simulink model "model_free"  (R2024a)
settings: Solver=FixedStepAuto  StartTime=0.0  StopTime=10.0  RelTol=1e-3
model workspace (MAT data in the model file):
  D = 0.006
  I = 0.04472
  Kp = 150
  Kpc = 250
  Kpp = 1600
  N = 17
  Nd = 10
  P = 5000
  Td = 0.005075
  Ti = 1000000
  Ts = 0.005
  alpha = 0.9
undefined symbols (not defined in the file or in its folder): GS, PID
libraries: slpidlib x3, simulink x2
settings Model: Creator=Henrique Mesquita  LastModifiedBy=Henrique Mesquita
settings SolverCC: ConcurrentTasks=on  PositivePriorityOrder=on
settings OptimizationCC: BlockReduction=off  OptimizeBlockIOStorage=off  ReuseModelBlockBuffer=off
settings DebuggingCC: TasksWithSamePriorityMsg=none  UnconnectedInputMsg=warning  UnconnectedOutputMsg=warning  UnconnectedLineMsg=warning
settings HardwareCC: ProdBitPerLong=64  ProdLongLongMode=on  ProdHWDeviceType=Intel->x86-64 (Linux 64)
settings ModelReferenceCC: EnableRefExpFcnMdlSchedulingChecks=on
settings RTWCC: Description=Speedgoat Real-Time Target Machine  SystemTargetFile=speedgoat.tlc  TemplateMakefile=slrealtime_default_tmf  Toolchain=Simulink Real-Time Toolchain  BuildConfiguration=Faster Runs  CodeExecutionProfiling=on  TargetLang=C++  GPUComputeCapability=3.5  DLArmComputeVersion=19.05
settings SimulinkRealTimeTargetCC: InstructionSetFMA=off  LogToMDFFile=off

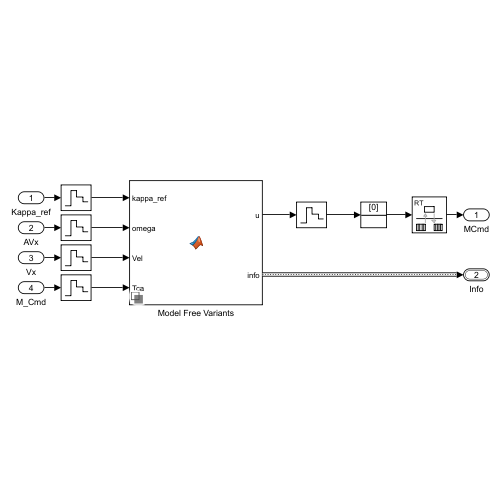
[thumbnail: Simulink's stored preview of the top-level diagram]
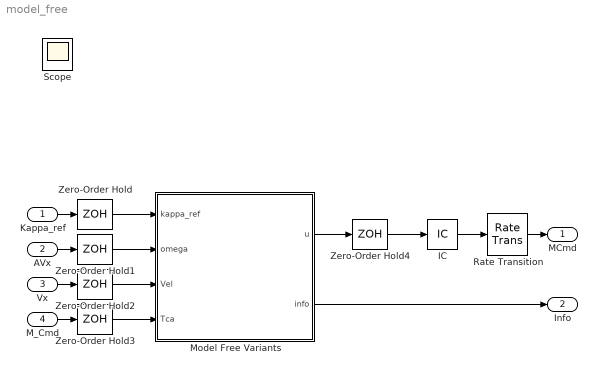
== system model_free ==
  Kappa_ref : Inport
  AVx : Inport  Port=2
  Vx : Inport  Port=3
  M_Cmd : Inport  Port=4
  IC : InitialCondition  Value=0
  Model Free Variants : Subsystem  Variant=on  VariantControlMode=label  VariantControl=Choice  LabelModeActiveChoice=MFC sliding window
  Rate Transition : RateTransition
  Zero-Order Hold{,1..4} (5 alike) : ZeroOrderHold  SampleTime=Ts
  MCmd : Outport
  Info : Outport  Port=2  OutDataTypeStr=Bus: control_info_bus
  Scope : Scope
  wires:
  AVx/1 -> Zero-Order Hold1/1
  IC/1 -> Rate Transition/1
  Vx/1 -> Zero-Order Hold2/1
  M_Cmd/1 -> Zero-Order Hold3/1
  Rate Transition/1 -> MCmd/1
  Kappa_ref/1 -> Zero-Order Hold/1
  Zero-Order Hold4/1 -> IC/1
  Zero-Order Hold/1 -> Model Free Variants/1(kappa_ref)
  Zero-Order Hold1/1 -> Model Free Variants/2(omega)
  Zero-Order Hold2/1 -> Model Free Variants/3(Vel)
  Zero-Order Hold3/1 -> Model Free Variants/4(Tca)
  Model Free Variants/1(u) -> Zero-Order Hold4/1
  Model Free Variants/2(info) -> Info/1

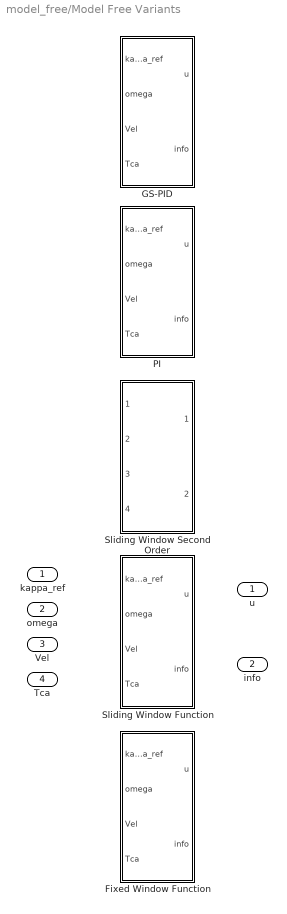
== system model_free/Model Free Variants ==
  kappa_ref : Inport
  omega : Inport  Port=2
  Vel : Inport  Port=3
  Tca : Inport  Port=4
  Fixed Window Function : MATLAB Function  TreatAsAtomicUnit=on  VariantControl=Choice_2
  GS-PID : Subsystem  VariantControl=GS-PID
  PI : Subsystem  VariantControl=PID
  Sliding Window Function : MATLAB Function  TreatAsAtomicUnit=on  VariantControl=MFC sliding window
  Sliding Window Second Order : ModelReference  ModelNameDialog=Sliding_Window_Second_Order  SimulationMode=Normal  VariantControl=Choice  ModelReferenceVersion=1.164
  u : Outport
  info : Outport  Port=2

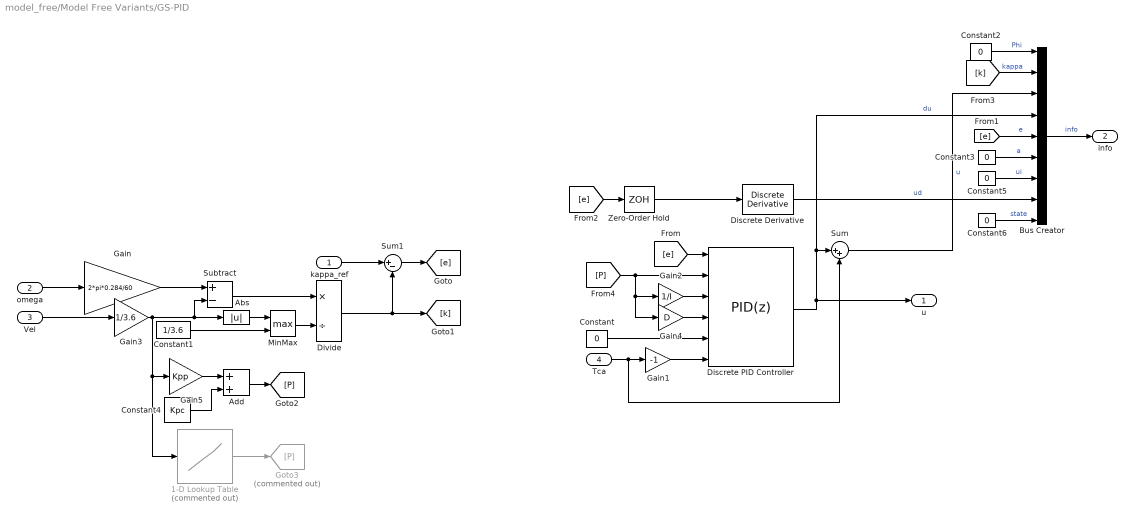
== system model_free/Model Free Variants/GS-PID ==
  kappa_ref : Inport
  omega : Inport  Port=2
  Vel : Inport  Port=3
  Tca : Inport  Port=4
  1-D Lookup Table : Lookup_n-D  Commented=on  NumberOfTableDimensions=1  BreakpointsForDimension1=[0:2]  Table=[Kpc,Kpc,Kpc+Kpp]  InternalRulePriority=Speed  RndMeth=Simplest
  Abs : Abs  SaturateOnIntegerOverflow=off
  Add : Sum
  Bus Creator : BusCreator  Inputs=9  OutDataTypeStr=Bus: control_info_bus
      settings: InheritFromInputs=off
  Constant{,2..3,5..6} (5 alike) : Constant  Value=0  SampleTime=Ts
  Constant1 : Constant  Value=1/3.6
  Constant4 : Constant  Value=Kpc
  Discrete Derivative : simulink/Discrete/Discrete Derivative  gainval=P*D  ICPrevScaledInput=0.0  OutMin=[]  OutMax=[]  OutDataType=fixdt(1, 16)  OutScaling=2^-10  DoSatur=off
  Discrete PID Controller : slpidlib/PID Controller  Controller=PID  Form=Parallel  TimeDomain=Discrete-time  UseExternalTs=off  SampleTime=Ts  IntegratorMethod=Trapezoidal  FilterMethod=Forward Euler  ControllerParametersSource=external  P=P  I=P/I  UseKiTs=off  D=P*D  UseExternalDerivativeSource=off  N=100  UseFilter=off  TunerSelectOption=Transfer Function Based (PID Tuner App)  InitialConditionSource=internal  InitialConditionForIntegrator=0  InitialConditionForFilter=0  DifferentiatorICPrevScaledInput=0  ExternalReset=none  TrackingMode=off  Kt=1  LimitOutput=on  SatLimitsSource=external  UpperSaturationLimit=inf  LowerSaturationLimit=-inf  LinearizeAsGain=off  AntiWindupMode=clamping  Kb=1  LimitIntegrator=off  UpperIntegratorSaturationLimit=inf  LowerIntegratorSaturationLimit=-inf  POutMin=[]  POutMax=[]  IOutMin=[]  IOutMax=[]  DOutMin=[]  DOutMax=[]  NOutMin=[]  NOutMax=[]  SumOutMin=[]  SumOutMax=[]  SaturationOutMin=[]  SaturationOutMax=[]  PParamMin=[]  PParamMax=[]  IParamMin=[]  IParamMax=[]  DParamMin=[]  DParamMax=[]  NParamMin=[]  NParamMax=[]  KbParamMin=[]  KbParamMax=[]  KtParamMin=[]  KtParamMax=[]  KbOutMin=[]  KbOutMax=[]  KtOutMin=[]  KtOutMax=[]  IntegratorOutMin=[]  IntegratorOutMax=[]  FilterOutMin=[]  FilterOutMax=[]  SumI1OutMin=[]  SumI1OutMax=[]  SumI2OutMin=[]  SumI2OutMax=[]  SumI3OutMin=[]  SumI3OutMax=[]  SumI4OutMin=[]  SumI4OutMax=[]  SumDOutMin=[]  SumDOutMax=[]  DifferentiatorOutMin=[]  DifferentiatorOutMax=[]  FilterDiffOutCoefMin=[]  FilterDiffOutCoefMax=[]  ReciprocalOutMin=[]  ReciprocalOutMax=[]  SumDenOutMin=[]  SumDenOutMax=[]  SumNumOutMin=[]  SumNumOutMax=[]  DivideOutMin=[]  DivideOutMax=[]  UdiffTsProdOutMin=[]  UdiffTsProdOutMax=[]  NTsProdOutMin=[]  NTsProdOutMax=[]  UintegralTsProdOutMin=[]  UintegralTsProdOutMax=[]  UngainTsProdOutMin=[]  UngainTsProdOutMax=[]  ClampingZeroOutDataTypeStr=Inherit: Inherit via back propagation  ClampingZeroOutMin=[]  ClampingZeroOutMax=[]  FilterDenConstantOutDataTypeStr=Inherit: Inherit via back propagation  FilterDenConstantOutMin=[]  FilterDenConstantOutMax=[]  PCopyOutDataTypeStr=Inherit: Inherit via back propagation  PCopyOutMin=[]  PCopyOutMax=[]  NCopyOutDataTypeStr=Inherit: Inherit via back propagation  NCopyOutMin=[]  NCopyOutMax=[]  IntegratorContinuousStateAttributes=''  IntegratorStateMustResolveToSignalObject=off  IntegratorRTWStateStorageClass=Auto  FilterContinuousStateAttributes=''  FilterStateMustResolveToSignalObject=off  FilterRTWStateStorageClass=Auto  ParallelPVariant=ExternalParameters  IdealPVariant=Disabled  IVariant=ExternalParameters  DVariant=ExternalParameters  IntegratorVariant=Discrete  SatVariant=External  AWVariant=DiscClampingParallel  PCopyVariant=Disabled  TRVariant=Disabled  FdbkBlocksVariant=Feedback  IdealPFdbkVariant=Passthrough  SatFdbkVariant=Passthrough  DerivativeFilterVariant=Differentiator  NVariant=Passthrough  NCopyVariant=Disabled_SignalSpec  FilterICVariant=InternalICsDifferentiator  IntegratorICVariant=InternalICs  ExternalResetVariant=Disabled  TRSumVariant=Passthrough  SumFdbkVariant=Enabled  SumVariant=Sum_PID  TsampFilterVariant=InternalTs  TsampNgainVariant=Passthrough  TsampIntegralVariant=Disabled_SignalSpec  ExternalSaturationOutDataTypeStr=Inherit: Same as second input  DerivativeSourceVariant=ErrorSignal
  Divide : Product  Inputs=*/
  Gain : Gain  Gain=2*pi*0.284/60
  Gain1 : Gain  Gain=-1
  Gain2 : Gain  Gain=1/I
  Gain3 : Gain  Gain=1/3.6
  Gain4 : Gain  Gain=D
  Gain5 : Gain  Gain=Kpp
  Goto3 : Goto  Commented=on  GotoTag=P
  MinMax : MinMax  Function=max  Inputs=2
  Subtract : Sum  Inputs=+-
  Sum : Sum  Inputs=|++
  Sum1 : Sum  Inputs=|+-
  Zero-Order Hold : ZeroOrderHold  SampleTime=Ts
  u : Outport
  info : Outport  Port=2
  wires:
  omega/1 -> Gain/1
  Gain/1 -> Subtract/1
  Vel/1 -> Gain3/1
  Subtract/1 -> Divide/1
  MinMax/1 -> Divide/2
  Constant1/1 -> MinMax/2
  Abs/1 -> MinMax/1
  Gain1/1 -> Discrete PID Controller/6
  Tca/1 -> Sum/2, Gain1/1
  Discrete PID Controller/1 -> u/1, Bus Creator/4, Sum/1  "du"
  Sum/1 -> Bus Creator/3  "u"
  Sum1/1 -> [e]
  Divide/1 -> [k], Sum1/2
  kappa_ref/1 -> Sum1/1
  Bus Creator/1 -> info/1  "info"
  Constant2/1 -> Bus Creator/1  "Phi"
  Gain3/1 -> 1-D Lookup Table/1, Gain5/1, Subtract/2, Abs/1
  Constant/1 -> Discrete PID Controller/5
  Discrete Derivative/1 -> Bus Creator/8  "ud"
  Zero-Order Hold/1 -> Discrete Derivative/1
  [e] -> Discrete PID Controller/1
  [e] -> Bus Creator/5  "e"
  [k] -> Bus Creator/2  "kappa"
  [e] -> Zero-Order Hold/1
  Gain2/1 -> Discrete PID Controller/3
  Gain4/1 -> Discrete PID Controller/4
  Gain5/1 -> Add/1
  Constant4/1 -> Add/2
  Add/1 -> [P]
  [P] -> Gain4/1, Gain2/1, Discrete PID Controller/2
  Constant3/1 -> Bus Creator/6  "a"
  Constant6/1 -> Bus Creator/9  "state"
  Constant5/1 -> Bus Creator/7  "ui"
  1-D Lookup Table/1 -> Goto3/1

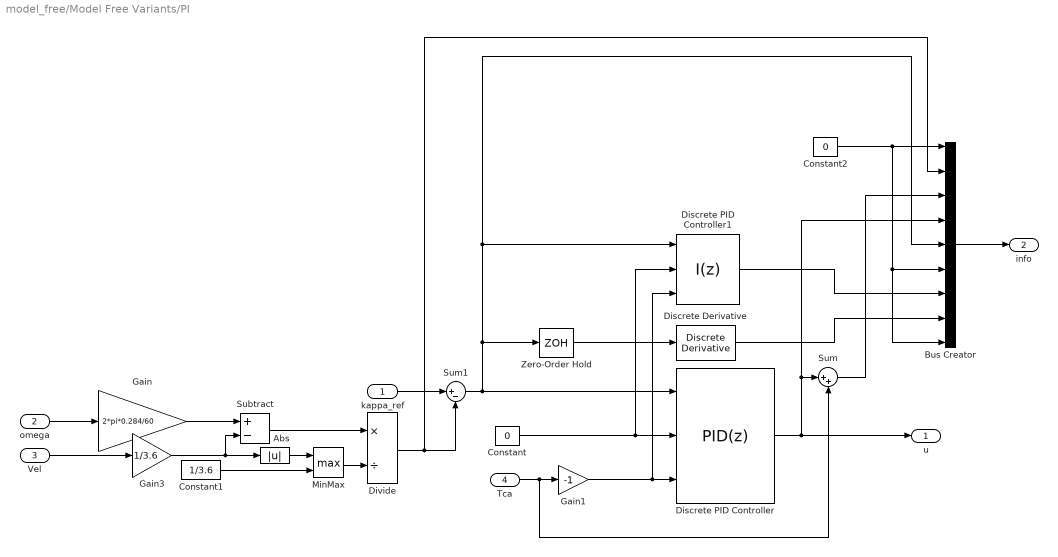
== system model_free/Model Free Variants/PI ==
  kappa_ref : Inport
  omega : Inport  Port=2
  Vel : Inport  Port=3
  Tca : Inport  Port=4
  Abs : Abs  SaturateOnIntegerOverflow=off
  Bus Creator : BusCreator  Inputs=9  OutDataTypeStr=Bus: control_info_bus
      settings: InheritFromInputs=off
  Constant : Constant  Value=0  SampleTime=Ts
  Constant1 : Constant  Value=1/3.6
  Constant2 : Constant  Value=0  SampleTime=Ts
  Discrete Derivative : simulink/Discrete/Discrete Derivative  gainval=P*D  ICPrevScaledInput=0.0  OutMin=[]  OutMax=[]  OutDataType=fixdt(1, 16)  OutScaling=2^-10  DoSatur=off
  Discrete PID Controller : slpidlib/PID Controller  Controller=PID  Form=Parallel  TimeDomain=Discrete-time  UseExternalTs=off  SampleTime=Ts  IntegratorMethod=Trapezoidal  FilterMethod=Forward Euler  ControllerParametersSource=internal  P=P  I=P/I  UseKiTs=off  D=P*D  UseExternalDerivativeSource=off  N=100  UseFilter=off  TunerSelectOption=Transfer Function Based (PID Tuner App)  InitialConditionSource=internal  InitialConditionForIntegrator=0  InitialConditionForFilter=0  DifferentiatorICPrevScaledInput=0  ExternalReset=none  TrackingMode=off  Kt=1  LimitOutput=on  SatLimitsSource=external  UpperSaturationLimit=inf  LowerSaturationLimit=-inf  LinearizeAsGain=off  AntiWindupMode=clamping  Kb=1  LimitIntegrator=off  UpperIntegratorSaturationLimit=inf  LowerIntegratorSaturationLimit=-inf  POutMin=[]  POutMax=[]  IOutMin=[]  IOutMax=[]  DOutMin=[]  DOutMax=[]  NOutMin=[]  NOutMax=[]  SumOutMin=[]  SumOutMax=[]  SaturationOutMin=[]  SaturationOutMax=[]  PParamMin=[]  PParamMax=[]  IParamMin=[]  IParamMax=[]  DParamMin=[]  DParamMax=[]  NParamMin=[]  NParamMax=[]  KbParamMin=[]  KbParamMax=[]  KtParamMin=[]  KtParamMax=[]  KbOutMin=[]  KbOutMax=[]  KtOutMin=[]  KtOutMax=[]  IntegratorOutMin=[]  IntegratorOutMax=[]  FilterOutMin=[]  FilterOutMax=[]  SumI1OutMin=[]  SumI1OutMax=[]  SumI2OutMin=[]  SumI2OutMax=[]  SumI3OutMin=[]  SumI3OutMax=[]  SumI4OutMin=[]  SumI4OutMax=[]  SumDOutMin=[]  SumDOutMax=[]  DifferentiatorOutMin=[]  DifferentiatorOutMax=[]  FilterDiffOutCoefMin=[]  FilterDiffOutCoefMax=[]  ReciprocalOutMin=[]  ReciprocalOutMax=[]  SumDenOutMin=[]  SumDenOutMax=[]  SumNumOutMin=[]  SumNumOutMax=[]  DivideOutMin=[]  DivideOutMax=[]  UdiffTsProdOutMin=[]  UdiffTsProdOutMax=[]  NTsProdOutMin=[]  NTsProdOutMax=[]  UintegralTsProdOutMin=[]  UintegralTsProdOutMax=[]  UngainTsProdOutMin=[]  UngainTsProdOutMax=[]  ClampingZeroOutDataTypeStr=Inherit: Inherit via back propagation  ClampingZeroOutMin=[]  ClampingZeroOutMax=[]  FilterDenConstantOutDataTypeStr=Inherit: Inherit via back propagation  FilterDenConstantOutMin=[]  FilterDenConstantOutMax=[]  PCopyOutDataTypeStr=Inherit: Inherit via back propagation  PCopyOutMin=[]  PCopyOutMax=[]  NCopyOutDataTypeStr=Inherit: Inherit via back propagation  NCopyOutMin=[]  NCopyOutMax=[]  IntegratorContinuousStateAttributes=''  IntegratorStateMustResolveToSignalObject=off  IntegratorRTWStateStorageClass=Auto  FilterContinuousStateAttributes=''  FilterStateMustResolveToSignalObject=off  FilterRTWStateStorageClass=Auto  ParallelPVariant=InternalParameters  IdealPVariant=Disabled  IVariant=InternalParameters  DVariant=InternalParameters  IntegratorVariant=Discrete  SatVariant=External  AWVariant=DiscClampingParallel  PCopyVariant=Disabled  TRVariant=Disabled  FdbkBlocksVariant=Feedback  IdealPFdbkVariant=Passthrough  SatFdbkVariant=Passthrough  DerivativeFilterVariant=Differentiator  NVariant=Passthrough  NCopyVariant=Disabled_SignalSpec  FilterICVariant=InternalICsDifferentiator  IntegratorICVariant=InternalICs  ExternalResetVariant=Disabled  TRSumVariant=Passthrough  SumFdbkVariant=Enabled  SumVariant=Sum_PID  TsampFilterVariant=InternalTs  TsampNgainVariant=Passthrough  TsampIntegralVariant=Disabled_SignalSpec  ExternalSaturationOutDataTypeStr=Inherit: Same as second input  DerivativeSourceVariant=ErrorSignal
  Discrete PID Controller1 : slpidlib/PID Controller  Controller=I  Form=Ideal  TimeDomain=Discrete-time  UseExternalTs=off  SampleTime=Ts  IntegratorMethod=Trapezoidal  FilterMethod=Forward Euler  ControllerParametersSource=internal  P=1  I=P/I  UseKiTs=off  D=0  UseExternalDerivativeSource=off  N=100  UseFilter=on  TunerSelectOption=Transfer Function Based (PID Tuner App)  InitialConditionSource=internal  InitialConditionForIntegrator=0  InitialConditionForFilter=0  DifferentiatorICPrevScaledInput=0  ExternalReset=none  TrackingMode=off  Kt=1  LimitOutput=on  SatLimitsSource=external  UpperSaturationLimit=inf  LowerSaturationLimit=-inf  LinearizeAsGain=off  AntiWindupMode=clamping  Kb=1  LimitIntegrator=off  UpperIntegratorSaturationLimit=inf  LowerIntegratorSaturationLimit=-inf  POutMin=[]  POutMax=[]  IOutMin=[]  IOutMax=[]  DOutMin=[]  DOutMax=[]  NOutMin=[]  NOutMax=[]  SumOutMin=[]  SumOutMax=[]  SaturationOutMin=[]  SaturationOutMax=[]  PParamMin=[]  PParamMax=[]  IParamMin=[]  IParamMax=[]  DParamMin=[]  DParamMax=[]  NParamMin=[]  NParamMax=[]  KbParamMin=[]  KbParamMax=[]  KtParamMin=[]  KtParamMax=[]  KbOutMin=[]  KbOutMax=[]  KtOutMin=[]  KtOutMax=[]  IntegratorOutMin=[]  IntegratorOutMax=[]  FilterOutMin=[]  FilterOutMax=[]  SumI1OutMin=[]  SumI1OutMax=[]  SumI2OutMin=[]  SumI2OutMax=[]  SumI3OutMin=[]  SumI3OutMax=[]  SumI4OutMin=[]  SumI4OutMax=[]  SumDOutMin=[]  SumDOutMax=[]  DifferentiatorOutMin=[]  DifferentiatorOutMax=[]  FilterDiffOutCoefMin=[]  FilterDiffOutCoefMax=[]  ReciprocalOutMin=[]  ReciprocalOutMax=[]  SumDenOutMin=[]  SumDenOutMax=[]  SumNumOutMin=[]  SumNumOutMax=[]  DivideOutMin=[]  DivideOutMax=[]  UdiffTsProdOutMin=[]  UdiffTsProdOutMax=[]  NTsProdOutMin=[]  NTsProdOutMax=[]  UintegralTsProdOutMin=[]  UintegralTsProdOutMax=[]  UngainTsProdOutMin=[]  UngainTsProdOutMax=[]  ClampingZeroOutDataTypeStr=Inherit: Inherit via back propagation  ClampingZeroOutMin=[]  ClampingZeroOutMax=[]  FilterDenConstantOutDataTypeStr=Inherit: Inherit via back propagation  FilterDenConstantOutMin=[]  FilterDenConstantOutMax=[]  PCopyOutDataTypeStr=Inherit: Inherit via back propagation  PCopyOutMin=[]  PCopyOutMax=[]  NCopyOutDataTypeStr=Inherit: Inherit via back propagation  NCopyOutMin=[]  NCopyOutMax=[]  IntegratorContinuousStateAttributes=''  IntegratorStateMustResolveToSignalObject=off  IntegratorRTWStateStorageClass=Auto  FilterContinuousStateAttributes=''  FilterStateMustResolveToSignalObject=off  FilterRTWStateStorageClass=Auto  ParallelPVariant=Disabled  IdealPVariant=Disabled  IVariant=InternalParameters  DVariant=Disabled  IntegratorVariant=Discrete  SatVariant=External  AWVariant=DiscClampingIdeal  PCopyVariant=Disabled  TRVariant=Disabled  FdbkBlocksVariant=Feedback  IdealPFdbkVariant=Passthrough  SatFdbkVariant=Passthrough  DerivativeFilterVariant=Disabled  NVariant=Disabled  NCopyVariant=Disabled_SignalSpec  FilterICVariant=Disabled  IntegratorICVariant=InternalICs  ExternalResetVariant=Disabled  TRSumVariant=Passthrough  SumFdbkVariant=Passthrough  SumVariant=Passthrough_I  TsampFilterVariant=InternalTs  TsampNgainVariant=Passthrough  TsampIntegralVariant=Disabled_SignalSpec  ExternalSaturationOutDataTypeStr=Inherit: Same as second input  DerivativeSourceVariant=Disabled
  Divide : Product  Inputs=*/
  Gain : Gain  Gain=2*pi*0.284/60
  Gain1 : Gain  Gain=-1
  Gain3 : Gain  Gain=1/3.6
  MinMax : MinMax  Function=max  Inputs=2
  Subtract : Sum  Inputs=+-
  Sum : Sum  Inputs=|++
  Sum1 : Sum  Inputs=|+-
  Zero-Order Hold : ZeroOrderHold  SampleTime=Ts
  u : Outport
  info : Outport  Port=2
  wires:
  omega/1 -> Gain/1
  Gain/1 -> Subtract/1
  Vel/1 -> Gain3/1
  Subtract/1 -> Divide/1
  MinMax/1 -> Divide/2
  Constant1/1 -> MinMax/2
  Abs/1 -> MinMax/1
  Gain1/1 -> Discrete PID Controller1/3, Discrete PID Controller/3
  Tca/1 -> Sum/2, Gain1/1
  Discrete PID Controller/1 -> u/1, Bus Creator/4, Sum/1
  Sum/1 -> Bus Creator/3
  Sum1/1 -> Zero-Order Hold/1, Bus Creator/5, Discrete PID Controller1/1, Discrete PID Controller/1
  Divide/1 -> Bus Creator/2, Sum1/2
  kappa_ref/1 -> Sum1/1
  Bus Creator/1 -> info/1
  Constant2/1 -> Bus Creator/9, Bus Creator/6, Bus Creator/1
  Discrete PID Controller1/1 -> Bus Creator/7
  Gain3/1 -> Subtract/2, Abs/1
  Constant/1 -> Discrete PID Controller1/2, Discrete PID Controller/2
  Discrete Derivative/1 -> Bus Creator/8
  Zero-Order Hold/1 -> Discrete Derivative/1

== matlab function model_free/Model Free Variants/Sliding Window Function ==
  data: kappa_ref input; u output; omega input; Vel input; Tca input; info output Bus: control_info_bus; Kp parameter; Td parameter; Ts parameter; alpha parameter; N parameter; Nd parameter
function [u,info] = fcn(kappa_ref, omega, Vel, Tca, Kp, Td, Ts, alpha, N, Nd)

%%% Definition of persistent variables
persistent u_mem;
persistent kappa_mem;
persistent k_ref_ant;
persistent k_ref_ant_ant;
persistent ud_ant;
persistent phi;
persistent alpha_chap;
persistent s_y;
persistent s_u;

%%% Initialization of the persistent values
if (isempty(u_mem)||isempty(kappa_mem)||isempty(k_ref_ant)||isempty(phi)||isempty(alpha_chap)||isempty(s_y)||isempty(s_u))
    
    %%% Initial allocation of the persistent variables
    phi = 0;
    alpha_chap = alpha;
    u_mem = zeros(1,N+1);
    kappa_mem = zeros(1,N+1);
    k_ref_ant = kappa_ref;
    k_ref_ant_ant = kappa_ref;
    ud_ant = 0;
    
    %%% Early calculation and saving of the algebraic estimator coefficients
    T = N*Ts;
    i = N-1:-1:1;
    s_y = -6/T^3*[Ts/2*(T-2*N*Ts), Ts*(T-2*i*Ts), Ts/2*(T-2*0*Ts)];
    s_u = -6/T^3*[Ts/2*(T-N*Ts)*(N*Ts), Ts*(T-i*Ts).*(i*Ts), Ts/2*(T-0*Ts)*(0*Ts)];
end

%%% Parameter transformations and definitions
omega = omega*2*pi/60;
Vel = Vel/3.6;
re = 0.284;
Iw = 0.8;

%%% Slip and error estimation
dot_yd = (kappa_ref - k_ref_ant) / Ts;
% dot_yd = (3*kappa_ref - 4*k_ref_ant+k_ref_ant_ant) / (2*Ts);
kappa = (omega*re-Vel)/(max([abs(Vel) 1/3.6]));
e = kappa-kappa_ref;

%%% Control signal calculation
% ud = Kp*Td/Ts*(kappa-kappa_mem(1));
% % ud = Td/(Td+Nd*Ts)*ud_ant + Kp*Nd*Td/(Td+Nd*Ts)*(kappa-kappa_mem(1));
% du = (-phi+dot_yd-Kp*e-ud)/alpha_chap;
ud = 0;
du = (-phi+dot_yd-Kp*e)/alpha_chap;

%%% Saturation of the control signal
if(du>0)
    du = 0;
elseif (du<-Tca)
    du = -Tca;
end

%%% Block outputs
% u = du+Tca;
u = du;
info = struct('Phi',phi,'kappa',kappa,'u',du+Tca,'du',du,'e',e,'a',alpha_chap,'ui',0,'ud',ud,'state',0);

%%% Memory actualization
for i = 0:N-1
    u_mem(N+1-i) = u_mem(N-i);
    kappa_mem(N+1-i) = kappa_mem(N-i);
end
u_mem(1) = du;
kappa_mem(1) = kappa;
k_ref_ant_ant = k_ref_ant;
k_ref_ant = kappa_ref;
ud_ant = ud;
alpha_chap = max([0.01,min([alpha,re/(Iw*max([0.001,abs(Vel)]))])]);
% alpha_chap = re/(Iw*(abs(Vel)+re/(Iw*alpha)));
% alpha_chap = alpha;

%%% Algebraic Estimation
phi=0;
for i=1:N+1
    phi = phi + s_y(i)*kappa_mem(i) + alpha_chap*s_u(i)*u_mem(i);
end

== matlab function model_free/Model Free Variants/Fixed Window Function ==
  data: kappa_ref input; u output; omega input; Vel input; Tca input; info output Bus: control_info_bus; Kp parameter; Ti parameter; Td parameter; Ts parameter; alpha parameter; N parameter; Nd parameter
function [u,info] = fcn(kappa_ref, omega, Vel, Tca, Kp, Ti, Td, Ts, alpha, N, Nd)

persistent n;
persistent u_ant;
persistent ui_ant;
persistent e_ant;
persistent kappa_ant;
persistent phi;
persistent phi_calc;

if (isempty(n)||isempty(u_ant)||isempty(ui_ant)||isempty(e_ant)||isempty(kappa_ant)||isempty(phi))
    n = 0;
    ui_ant = 0;
    e_ant = 0;
    phi = 0;
    phi_calc = 0;
    a = 0;
    u_ant = 0;
    kappa_ant = 0;
end

omega = omega*2*pi/60;
Vel = Vel/3.6;
re = 0.284;

dot_yd = 0;
% if (omega*re >= Vel)
%     kappa = (omega*re-Vel)/(omega*re+1);
% else
%     kappa = (omega*re-Vel)/(Vel+1);
% end
kappa = (omega*re-Vel)/(max([Vel 4/3.6]));
e = kappa-kappa_ref;
T = N*Ts;

ui = Kp*Ts/(2*Ti)*(e+e_ant)+ui_ant;
% ui = 0;

if (abs(ui)>5)
    ui = sign(ui)*5;
end

% ud = Kp*Td/Ts*(e-e_ant);
ud = Kp*Td/Ts*(kappa-kappa_ant);
% ud = Td/(Td+Nd*Ts)*u_ant + Kp*Nd*Td/(Td+Nd*Ts)*(e-e_ant);
% ud = Td/(Td+Nd*Ts)*u_ant + Kp*Nd*Td/(Td+Nd*Ts)*(kappa-kappa_ant);
du = (-phi+dot_yd-Kp*e-ui-ud)/alpha;

% if(du>Tca)
%     du = Tca;
% elseif (du<0)
%     du = 0;
% end
% u = du;

if(du>0)
    du = 0;
elseif (du<-Tca)
    du = -Tca;
end
u = du+Tca;

info = struct('Phi',phi,'kappa',kappa,'u',u,'du',du,'e',e,'a',0,'ui',ui,'ud',ud,'state',0);

n = n+1;
phi_calc = phi_calc -6/T^3*(Ts/2*((T-2*n*Ts)*kappa+(T-2*(n-1)*Ts)*kappa_ant)+alpha*Ts/2*((T-n*Ts)*(n*Ts)*du+(T-(n-1)*Ts)*((n-1)*Ts)*u_ant));
if (n == N)
    phi = phi_calc;
    phi_calc = 0;
    n=0;
end


u_ant = du;
kappa_ant = kappa;
ui_ant = ui;
e_ant = e;
